simulink model "spacecraft_model"  (R2024a)
settings: Solver=VariableStepAuto  StartTime=0.0  StopTime=tstop  RelTol=1e-3
undefined symbols (not defined in the file or in its folder): dt, time_between_measurements
libraries: simulink x3, aerolibutil x1, mysharedTrackingLibrary x1, sharedTrackingLibrary x1, sharedutil x1
settings Model: Creator=brian  LastModifiedBy=jantonio
settings SolverCC: DecoupledContinuousIntegration=on
settings RTWCC: GPUComputeCapability=3.5

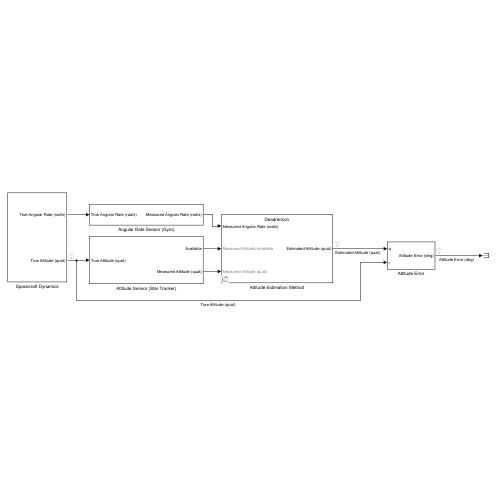
[thumbnail: Simulink's stored preview of the top-level diagram]
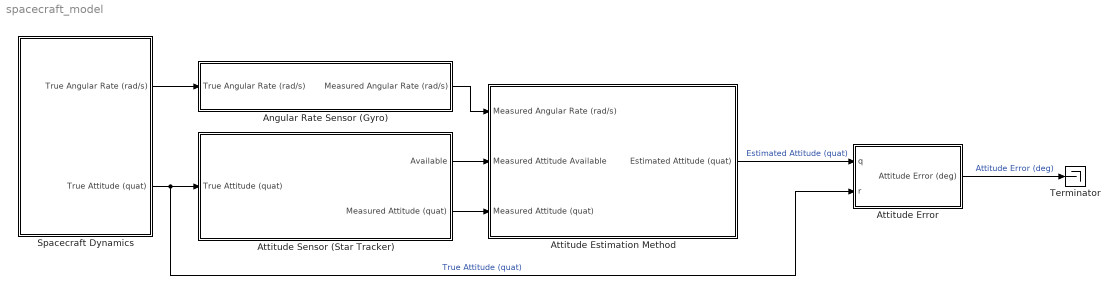
== system spacecraft_model ==
  Angular Rate Sensor (Gyro) : Subsystem
  Attitude Error : Subsystem
  Attitude Estimation Method : Subsystem  Variant=on
  Attitude Sensor (Star Tracker) : Subsystem
  Spacecraft Dynamics : Subsystem
  Terminator : Terminator
  wires:
  Spacecraft Dynamics/1(True Angular Rate (rad/s)) -> Angular Rate Sensor (Gyro)/1(True Angular Rate (rad/s))
  Spacecraft Dynamics/2(True Attitude (quat)) -> Attitude Error/2(r), Attitude Sensor (Star Tracker)/1(True Attitude (quat))  "True Attitude (quat)"
  Angular Rate Sensor (Gyro)/1(Measured Angular Rate (rad/s)) -> Attitude Estimation Method/1(Measured Angular Rate (rad/s))
  Attitude Estimation Method/1(Estimated Attitude (quat)) -> Attitude Error/1(q)  "Estimated Attitude (quat)"
  Attitude Sensor (Star Tracker)/1(Available) -> Attitude Estimation Method/2(Measured Attitude Available)
  Attitude Sensor (Star Tracker)/2(Measured Attitude (quat)) -> Attitude Estimation Method/3(Measured Attitude (quat))
  Attitude Error/1(Attitude Error (deg)) -> Terminator/1  "Attitude Error (deg)"

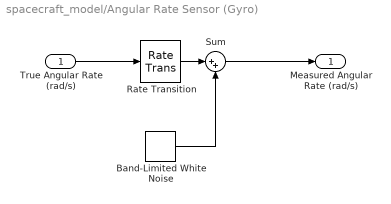
== system spacecraft_model/Angular Rate Sensor (Gyro) ==
  True Angular Rate (rad/s) : Inport
  Band-Limited White Noise : simulink/Sources/Band-Limited White Noise  Cov=gyro_noise  Ts=dt  seed=[1 2 3]
  Rate Transition : RateTransition  OutPortSampleTime=dt
  Sum : Sum  Inputs=|++
  Measured Angular Rate (rad/s) : Outport
  wires:
  Sum/1 -> Measured Angular Rate (rad/s)/1
  True Angular Rate (rad/s)/1 -> Rate Transition/1
  Rate Transition/1 -> Sum/1
  Band-Limited White Noise/1 -> Sum/2

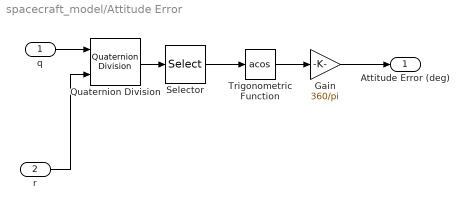
== system spacecraft_model/Attitude Error ==
  q : Inport
  r : Inport  Port=2
  Gain : Gain  Gain=360/pi
  Quaternion Division : aerolibutil/Quaternion Division
  Selector : Selector  InputPortWidth=4  IndexOptions=Index vector (dialog)  Indices=1  OutputSizes=1
  Trigonometric Function : Trigonometry  Operator=acos
  Attitude Error (deg) : Outport
  wires:
  Gain/1 -> Attitude Error (deg)/1
  Selector/1 -> Trigonometric Function/1
  Quaternion Division/1 -> Selector/1
  q/1 -> Quaternion Division/1
  r/1 -> Quaternion Division/2
  Trigonometric Function/1 -> Gain/1

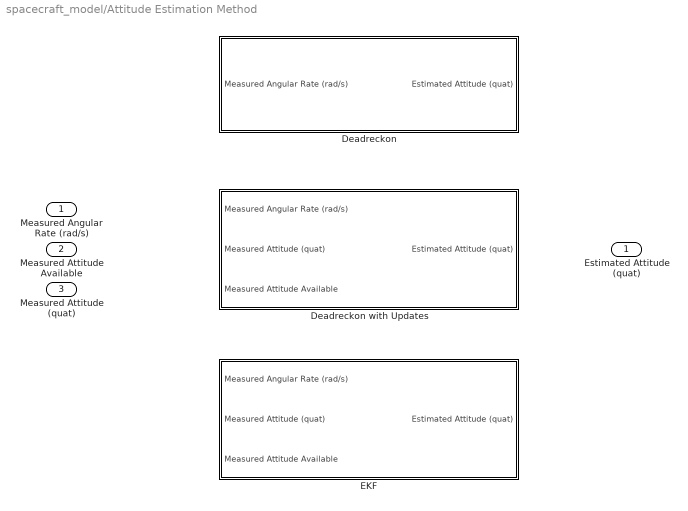
== system spacecraft_model/Attitude Estimation Method ==
  Measured Angular Rate (rad/s) : Inport
  Measured Attitude Available : Inport  Port=2
  Measured Attitude (quat) : Inport  Port=3
  Deadreckon : Subsystem  VariantControl=ad_method == 1
  Deadreckon with Updates : Subsystem  VariantControl=ad_method == 2
  EKF : Subsystem  VariantControl=ad_method == 3
  Estimated Attitude (quat) : Outport

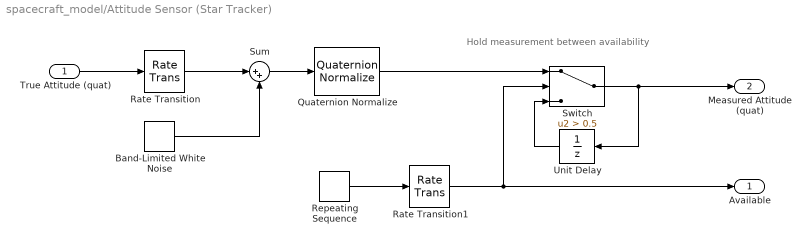
== system spacecraft_model/Attitude Sensor (Star Tracker) ==
  note: Hold measurement between availability
  True Attitude (quat) : Inport
  Band-Limited White Noise : simulink/Sources/Band-Limited White Noise  Cov=star_tracker_noise  Ts=dt  seed=[4 5 6 7]
  Quaternion Normalize : sharedutil/Quaternion Normalize  aMode=aMode
  Rate Transition : RateTransition  OutPortSampleTime=dt
  Rate Transition1 : RateTransition  OutPortSampleTime=dt
  Repeating Sequence : simulink/Sources/Repeating Sequence  rep_seq_t=[0, dt, time_between_measurements]  rep_seq_y=[1 0 0]
  Sum : Sum  Inputs=|++
  Switch : Switch  Criteria=u2 > Threshold  Threshold=0.5  SaturateOnIntegerOverflow=off  InputSameDT=off
  Unit Delay : UnitDelay  InitialCondition=[1 0 0 0]  SampleTime=-1  HasFrameUpgradeWarning=on
  Available : Outport
  Measured Attitude (quat) : Outport  Port=2
  wires:
  Band-Limited White Noise/1 -> Sum/2
  True Attitude (quat)/1 -> Rate Transition/1
  Rate Transition/1 -> Sum/1
  Switch/1 -> Unit Delay/1, Measured Attitude (quat)/1
  Sum/1 -> Quaternion Normalize/1
  Repeating Sequence/1 -> Rate Transition1/1
  Rate Transition1/1 -> Switch/2, Available/1
  Quaternion Normalize/1 -> Switch/1
  Unit Delay/1 -> Switch/3

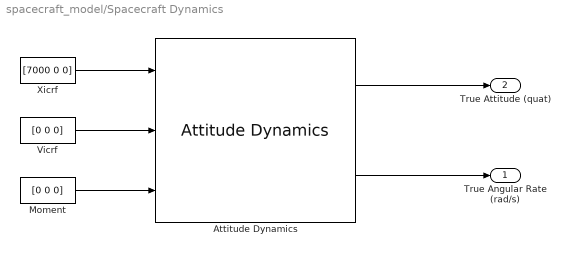
== system spacecraft_model/Spacecraft Dynamics ==
  Attitude Dynamics : AttitudeDynamics  stateFrame=Fixed-frame  dateOut=off  inertia=inertia_tensor_kg_m2  attitudeFrame=LVLH  attitude=initial_attitude_quat  attitudeRate=initial_rate_radps  units=Metric (km/s)  angleUnits=Radians
  Moment : Constant  Value=[0 0 0]
  Vicrf : Constant  Value=[0 0 0]
  Xicrf : Constant  Value=[7000 0 0]
  True Angular Rate (rad/s) : Outport
  True Attitude (quat) : Outport  Port=2
  wires:
  Attitude Dynamics/2 -> True Angular Rate (rad/s)/1
  Moment/1 -> Attitude Dynamics/3
  Attitude Dynamics/1 -> True Attitude (quat)/1
  Vicrf/1 -> Attitude Dynamics/2
  Xicrf/1 -> Attitude Dynamics/1

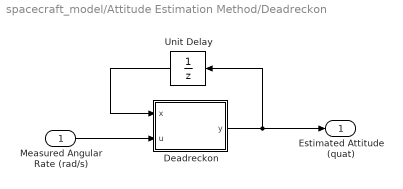
== system spacecraft_model/Attitude Estimation Method/Deadreckon ==
  Measured Angular Rate (rad/s) : Inport
  Deadreckon : MATLAB Function  TreatAsAtomicUnit=on
  Unit Delay : UnitDelay  InitialCondition=[1 0 0 0]'  SampleTime=-1  HasFrameUpgradeWarning=on
  Estimated Attitude (quat) : Outport
  wires:
  Deadreckon/1(y) -> Estimated Attitude (quat)/1, Unit Delay/1
  Measured Angular Rate (rad/s)/1 -> Deadreckon/2(u)
  Unit Delay/1 -> Deadreckon/1(x)

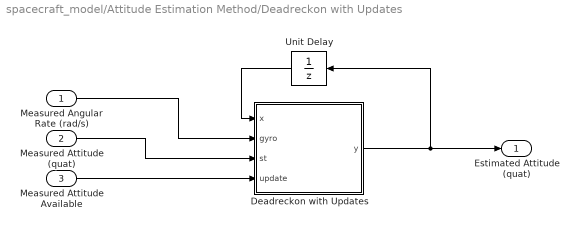
== system spacecraft_model/Attitude Estimation Method/Deadreckon with Updates ==
  Measured Angular Rate (rad/s) : Inport
  Measured Attitude (quat) : Inport  Port=2
  Measured Attitude Available : Inport  Port=3
  Deadreckon with Updates : MATLAB Function  TreatAsAtomicUnit=on
  Unit Delay : UnitDelay  InitialCondition=[1 0 0 0]'  SampleTime=-1  HasFrameUpgradeWarning=on
  Estimated Attitude (quat) : Outport
  wires:
  Measured Attitude (quat)/1 -> Deadreckon with Updates/3(st)
  Measured Angular Rate (rad/s)/1 -> Deadreckon with Updates/2(gyro)
  Unit Delay/1 -> Deadreckon with Updates/1(x)
  Deadreckon with Updates/1(y) -> Unit Delay/1, Estimated Attitude (quat)/1
  Measured Attitude Available/1 -> Deadreckon with Updates/4(update)

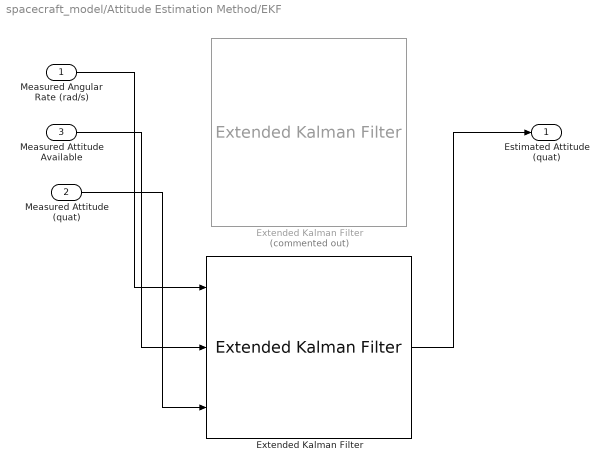
== system spacecraft_model/Attitude Estimation Method/EKF ==
  Measured Angular Rate (rad/s) : Inport
  Measured Attitude (quat) : Inport  Port=2
  Measured Attitude Available : Inport  Port=3
  Extended Kalman Filter : mysharedTrackingLibrary/Extended Kalman Filter  StateTransitionFcn=stateTransitionFnc  HasStateTransitionJacobianFcn=off  HasAdditiveProcessNoise=Additive  ProcessNoise=process_covariance  HasTimeVaryingProcessNoise=off  HasStateTransitionFcnExtraArgument=1  InitialState=initial_state  InitialStateCovariance=initial_covariance  MeasurementFcn1=measurementFnc  HasMeasurementJacobianFcn1=off  HasMeasurementEnablePort1=on  HasAdditiveMeasurementNoise1=Additive  MeasurementNoise1=measurement_covariance  HasTimeVaryingMeasurementNoise1=off  HasMeasurementFcnExtraArgument1=0  HasMeasurementWrapping1=off  HasMeasurementJacobianFcn2=off  HasMeasurementEnablePort2=off  HasAdditiveMeasurementNoise2=Additive  MeasurementNoise2=1  HasTimeVaryingMeasurementNoise2=off  HasMeasurementFcnExtraArgument2=0  HasMeasurementWrapping2=off  HasMeasurementJacobianFcn3=off  HasMeasurementEnablePort3=off  HasAdditiveMeasurementNoise3=Additive  MeasurementNoise3=1  HasTimeVaryingMeasurementNoise3=off  HasMeasurementFcnExtraArgument3=0  HasMeasurementWrapping3=off  HasMeasurementJacobianFcn4=off  HasMeasurementEnablePort4=off  HasAdditiveMeasurementNoise4=Additive  MeasurementNoise4=1  HasTimeVaryingMeasurementNoise4=off  HasMeasurementFcnExtraArgument4=0  HasMeasurementWrapping4=off  HasMeasurementJacobianFcn5=off  HasMeasurementEnablePort5=off  HasAdditiveMeasurementNoise5=Additive  MeasurementNoise5=1  HasTimeVaryingMeasurementNoise5=off  HasMeasurementFcnExtraArgument5=0  HasMeasurementWrapping5=off  EnableMultirate=off  StateTransitionFcnSampleTime=1  MeasurementFcn1SampleTime=1  MeasurementFcn2SampleTime=1  MeasurementFcn3SampleTime=1  MeasurementFcn4SampleTime=1  MeasurementFcn5SampleTime=1  UseCurrentEstimator=off  OutputStateCovariance=off  DataType=double  SampleTime=dt  NumberOfMeasurements=1
  "Extended Kalman Filter " : sharedTrackingLibrary/Extended Kalman Filter  Commented=on  StateTransitionFcn=stateTransitionFnc  HasStateTransitionJacobianFcn=off  HasAdditiveProcessNoise=Additive  ProcessNoise=process_covariance  HasTimeVaryingProcessNoise=off  HasStateTransitionFcnExtraArgument=1  InitialState=initial_state  InitialStateCovariance=initial_covariance  MeasurementFcn1=measurementFnc  HasMeasurementJacobianFcn1=off  HasMeasurementEnablePort1=on  HasAdditiveMeasurementNoise1=Additive  MeasurementNoise1=measurement_covariance  HasTimeVaryingMeasurementNoise1=off  HasMeasurementFcnExtraArgument1=0  HasMeasurementWrapping1=off  MeasurementFcn2=myMeasurementFcn  HasMeasurementJacobianFcn2=off  HasMeasurementEnablePort2=off  HasAdditiveMeasurementNoise2=Additive  MeasurementNoise2=1  HasTimeVaryingMeasurementNoise2=off  HasMeasurementFcnExtraArgument2=0  HasMeasurementWrapping2=off  MeasurementFcn3=myMeasurementFcn  HasMeasurementJacobianFcn3=off  HasMeasurementEnablePort3=off  HasAdditiveMeasurementNoise3=Additive  MeasurementNoise3=1  HasTimeVaryingMeasurementNoise3=off  HasMeasurementFcnExtraArgument3=0  HasMeasurementWrapping3=off  MeasurementFcn4=myMeasurementFcn  HasMeasurementJacobianFcn4=off  HasMeasurementEnablePort4=off  HasAdditiveMeasurementNoise4=Additive  MeasurementNoise4=1  HasTimeVaryingMeasurementNoise4=off  HasMeasurementFcnExtraArgument4=0  HasMeasurementWrapping4=off  MeasurementFcn5=myMeasurementFcn  HasMeasurementJacobianFcn5=off  HasMeasurementEnablePort5=off  HasAdditiveMeasurementNoise5=Additive  MeasurementNoise5=1  HasTimeVaryingMeasurementNoise5=off  HasMeasurementFcnExtraArgument5=0  HasMeasurementWrapping5=off  EnableMultirate=off  StateTransitionFcnSampleTime=0.01  MeasurementFcn1SampleTime=1  MeasurementFcn2SampleTime=1  MeasurementFcn3SampleTime=1  MeasurementFcn4SampleTime=1  MeasurementFcn5SampleTime=1  UseCurrentEstimator=off  OutputStateCovariance=off  DataType=double  SampleTime=dt  NumberOfMeasurements=1
  Estimated Attitude (quat) : Outport
  wires:
  Measured Angular Rate (rad/s)/1 -> Extended Kalman Filter/1
  Extended Kalman Filter/1 -> Estimated Attitude (quat)/1
  Measured Attitude (quat)/1 -> Extended Kalman Filter/3
  Measured Attitude Available/1 -> Extended Kalman Filter/2

== matlab function spacecraft_model/Attitude Estimation Method/Deadreckon with Updates/Deadreckon with Updates ==
  data: x input; gyro input; y output size=4; st input; update input
function y = fcn(x, gyro, st, update)

rotMat = 0.01/2*[-x(2), -x(3), -x(4);
                  x(1), -x(4),  x(3);
                  x(4),  x(1), -x(2);
                 -x(3),  x(2),  x(1)];

x = x + rotMat*[gyro(1), gyro(2), gyro(3)]';

y = x./norm(x);

if update
    y = st;
end

== matlab function spacecraft_model/Attitude Estimation Method/Deadreckon/Deadreckon ==
  data: x input; u input; y output size=4
function y = fcn(x, u)

rotMat = 0.01/2*[-x(2), -x(3), -x(4);
                  x(1), -x(4),  x(3);
                  x(4),  x(1), -x(2);
                 -x(3),  x(2),  x(1)];

x = x + rotMat*[u(1), u(2), u(3)]';

y = x./norm(x);
